simulink model "Surgical_RCM_Sim"  (R2026a)
settings: Solver=VariableStepAuto  StopTime=30.0
settings Model: Creator=shueb  LastModifiedBy=shueb

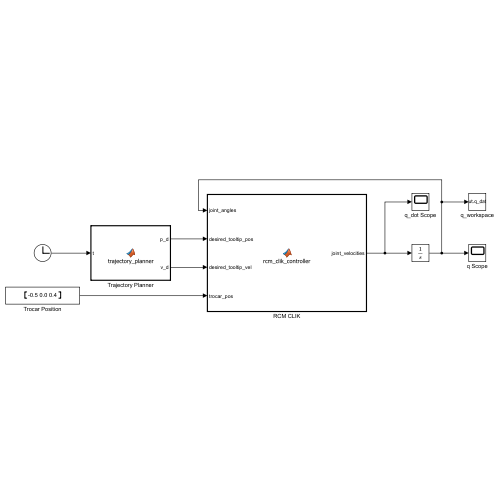
[thumbnail: Simulink's stored preview of the top-level diagram]
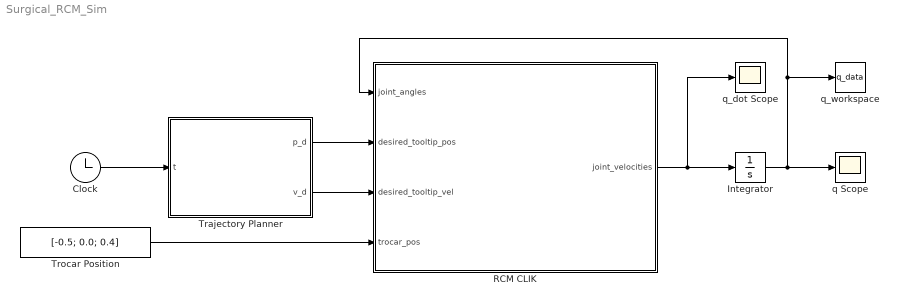
== system Surgical_RCM_Sim ==
  Clock : Clock
  Integrator : Integrator  InitialCondition=[0; 0.4085; 3.1416; 0.6128; -3.1416; 2.1203; 3.1416]
  RCM CLIK : MATLAB Function  TreatAsAtomicUnit=on
  Trajectory Planner : MATLAB Function  TreatAsAtomicUnit=on
  Trocar Position : Constant  Value=[-0.5; 0.0; 0.4]
  q Scope : Scope
  q_dot Scope : Scope
  q_workspace : ToWorkspace  VariableName=q_data  SampleTime=-1
  wires:
  Clock/1 -> Trajectory Planner/1(t)
  Trajectory Planner/1(p_d) -> RCM CLIK/2(desired_tooltip_pos)
  Trajectory Planner/2(v_d) -> RCM CLIK/3(desired_tooltip_vel)
  Trocar Position/1 -> RCM CLIK/4(trocar_pos)
  Integrator/1 -> RCM CLIK/1(joint_angles), q_workspace/1, q Scope/1
  RCM CLIK/1(joint_velocities) -> Integrator/1, q_dot Scope/1

== matlab function Surgical_RCM_Sim/RCM CLIK ==
  data: joint_angles input; joint_velocities output; desired_tooltip_pos input; desired_tooltip_vel input; trocar_pos input
function joint_velocities = rcm_clik_controller(joint_angles, desired_tooltip_pos, desired_tooltip_vel, trocar_pos)
    %#codegen
    assert(isa(joint_angles, 'double'));
    assert(all(size(joint_angles) == [7, 1]));
    assert(isa(desired_tooltip_pos, 'double'));
    assert(all(size(desired_tooltip_pos) == [3, 1]));
    assert(isa(desired_tooltip_vel, 'double'));
    assert(all(size(desired_tooltip_vel) == [3, 1]));
    assert(isa(trocar_pos, 'double'));
    assert(all(size(trocar_pos) == [3, 1]));

    joint_velocities = zeros(7, 1);
    
    % Controller Gains
    K_rcm = 10;
    K_tool = 20;
    
    % 1. Forward Kinematics (Flange Pose and Needle Orientation)
    flange_pose = kuka_direct_kinematics(joint_angles);
    flange_pos = flange_pose(1:3, 4);
    flange_rot = flange_pose(1:3, 1:3);
    needle_direction = flange_rot(:, 3); % Z-axis of the flange points along the needle
    
    % Flange Jacobians
    jacobian_flange = jacobian_kuka(joint_angles);
    flange_jac_linear = jacobian_flange(1:3, :);
    flange_jac_angular = jacobian_flange(4:6, :);
    
    % 2. Tool Kinematics (Tooltip Position and Jacobian)
    needle_length = 0.15; % 15 cm tool
    tooltip_pos = flange_pos + needle_length * needle_direction;
    
    skew_Lz = [0, -needle_length*needle_direction(3), needle_length*needle_direction(2);
               needle_length*needle_direction(3), 0, -needle_length*needle_direction(1);
               -needle_length*needle_direction(2), needle_length*needle_direction(1), 0];
    tooltip_jacobian = flange_jac_linear - skew_Lz * flange_jac_angular;
    
    % 3. RCM Kinematics (Trocar Constraint Error and Jacobian)
    insertion_depth = (trocar_pos - flange_pos)' * needle_direction;
    closest_point_on_shaft = flange_pos + insertion_depth * needle_direction;
    rcm_error = trocar_pos - closest_point_on_shaft;
    
    skew_lamz = [0, -insertion_depth*needle_direction(3), insertion_depth*needle_direction(2);
                 insertion_depth*needle_direction(3), 0, -insertion_depth*needle_direction(1);
                 -insertion_depth*needle_direction(2), insertion_depth*needle_direction(1), 0];
    closest_point_jacobian = flange_jac_linear - skew_lamz * flange_jac_angular;
    
    % Project Jacobian onto plane orthogonal to needle direction
    Proj_ortho = eye(3) - needle_direction * needle_direction';
    rcm_jacobian = Proj_ortho * closest_point_jacobian;
    
    % 4. Task-Priority Closed-Loop Inverse Kinematics (CLIK)
    
    % Task 1: RCM Trocar Constraint (Highest Priority)
    rcm_jacobian_pinv = pinv(rcm_jacobian);
    joint_vel_rcm = rcm_jacobian_pinv * (K_rcm * rcm_error);
    
    % Task 2: Tooltip Trajectory Tracking (Secondary Priority)
    tooltip_error = desired_tooltip_pos - tooltip_pos;
    tooltip_vel_from_rcm = tooltip_jacobian * joint_vel_rcm;
    tooltip_vel_required = desired_tooltip_vel + K_tool * tooltip_error - tooltip_vel_from_rcm;
    
    % Project tooltip tracking into RCM null-space to guarantee no trocar motion
    nullspace_projection = eye(7) - rcm_jacobian_pinv * rcm_jacobian;
    tooltip_jacobian_projected = tooltip_jacobian * nullspace_projection;
    
    % Damped Least Squares for Secondary Task to avoid singularities
    lambda_damp = 0.01;
    tooltip_jacobian_projected_pinv = tooltip_jacobian_projected' / (tooltip_jacobian_projected * tooltip_jacobian_projected' + lambda_damp^2 * eye(3));
    
    joint_vel_tooltip = tooltip_jacobian_projected_pinv * tooltip_vel_required;
    
    % Combine velocities
    joint_velocities = joint_vel_rcm + joint_vel_tooltip;
end

== matlab function Surgical_RCM_Sim/Trajectory Planner ==
  data: t input; p_d output; v_d output
function [p_d, v_d] = trajectory_planner(t)
    %#codegen
    assert(isa(t, 'double'));
    assert(all(size(t) == [1, 1]));
    
    p_d = zeros(3, 1);
    v_d = zeros(3, 1);
    
    % Reachable Targets (Trocar at [-0.5; 0.0; 0.4], L = 0.15m)
    m0 = [-0.50;  0.00; 0.30]; % Starting position
    m1 = [-0.50;  0.08; 0.28]; % Target 1
    m2 = [-0.52;  0.04; 0.27]; % Target 2 (Repositioned)
    m3 = [-0.46; -0.04; 0.32]; % Target 3 (Repositioned)
    m4 = [-0.50; -0.08; 0.28]; % Target 4
    m5 = [-0.55;  0.00; 0.30]; % Target 5
    
    T_seg = 5.0; % 5 seconds per segment
    
    if t < T_seg
        p_start = m0; p_end = m1;
        tau = t;
    elseif t < 2*T_seg
        p_start = m1; p_end = m2;
        tau = t - T_seg;
    elseif t < 3*T_seg
        p_start = m2; p_end = m3;
        tau = t - 2*T_seg;
    elseif t < 4*T_seg
        p_start = m3; p_end = m4;
        tau = t - 3*T_seg;
    elseif t < 5*T_seg
        p_start = m4; p_end = m5;
        tau = t - 4*T_seg;
    else
        p_start = m5; p_end = m5;
        tau = T_seg;
    end
    
    % Cubic polynomial s(tau) from 0 to 1
    if tau <= 0
        s = 0; s_dot = 0;
    elseif tau >= T_seg
        s = 1; s_dot = 0;
    else
        s = 3*(tau/T_seg)^2 - 2*(tau/T_seg)^3;
        s_dot = (6*tau/(T_seg^2)) - (6*tau^2/(T_seg^3));
    end
    
    p_d = p_start + (p_end - p_start) * s;
    v_d = (p_end - p_start) * s_dot;
end
